simulink subsystem "SimscapePlantModels"  (R2023a)
settings: Solver=VariableStepAuto  StartTime=0.0  StopTime=10.0  RelTol=1e-3
undefined symbols (not defined in the file): AxlFL, AxlFR, AxlRL, AxlRR, EM1, EM2, EM3, EM4, PlntDCDCVoltInit, PlntTrnsfrCaseAxlSpdLock, PlntTrnsfrCaseTrqSplitRatio, ThrmBatt, ThrmBatt1, ThrmBatt2, ThrmBatt3, ThrmBatt4, ThrmEM, ThrmEM1, ThrmEM2, ThrmEM3, ThrmEM4, ThrmPwrE
libraries: fl_lib x30, nesl_utility_internal x13, sdl_lib x3, nesl_utility x2, vehdynlibsens x1
(part 1 of 2)
settings Model: ModifiedByFormat=The MathWorks, Inc.  Creator=The MathWorks, Inc.  LastModifiedBy=The MathWorks, Inc.
settings SolverCC: MaxZcPerStep=1
settings OptimizationCC: ReuseModelBlockBuffer=off
settings DebuggingCC: UnconnectedInputMsg=warning  UnconnectedOutputMsg=warning  UnconnectedLineMsg=warning  SubsystemReferenceDiagnosticForUnitTest=warning
settings ModelReferenceCC: EnableRefExpFcnMdlSchedulingChecks=on
settings RTWCC: DLArmComputeVersion=19.05

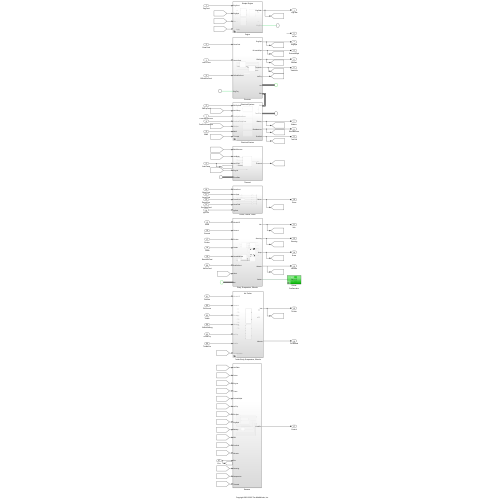
[thumbnail: Simulink's stored preview of the top-level diagram]
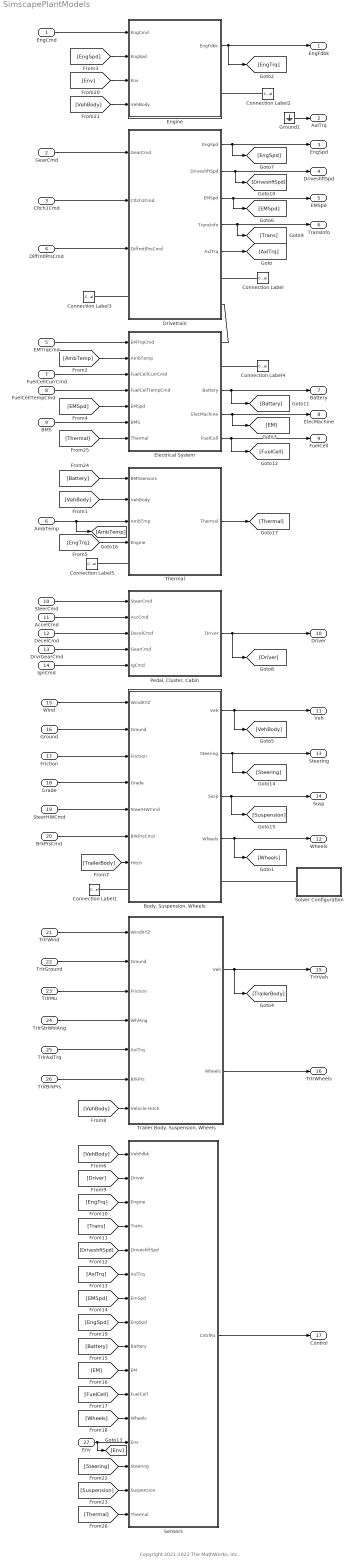
== system SimscapePlantModels ==
  note: Copyright 2021-2022 The MathWorks, Inc.
  EngCmd : Inport
  GearCmd : Inport  Port=2
  Cltch1Cmd : Inport  Port=3
  DiffrntlPrsCmd : Inport  Port=4
  EMTrqCmd : Inport  Port=5
  AmbTemp : Inport  Port=6
  FuelCellCurrCmd : Inport  Port=7
  FuelCellTempCmd : Inport  Port=8
  BMS : Inport  Port=9
  SteerCmd : Inport  Port=10
  AccelCmd : Inport  Port=11
  DecelCmd : Inport  Port=12
  DrvrGearCmd : Inport  Port=13
  IgnCmd : Inport  Port=14
  Wind : Inport  Port=15
  Ground : Inport  Port=16
  Friction : Inport  Port=17
  Grade : Inport  Port=18
  SteerHWCmd : Inport  Port=19
  BrkPrsCmd : Inport  Port=20
  TrlrWind : Inport  Port=21
  TrlrGround : Inport  Port=22
  TrlrMu : Inport  Port=23
  TrlrStrWhlAng : Inport  Port=24
  TrlrAxlTrq : Inport  Port=25
  TrlrBrkPrs : Inport  Port=26
  Env : Inport  Port=27
  "Body, Suspension, Wheels" : Subsystem  VariantControl=Longitudinal Vehicle Dynamics
  Connection Label : ConnectionLabel  Label=Axl
  Connection Label1 : ConnectionLabel  Label=Axl
  Connection Label2 : ConnectionLabel  Label=EngTrq
  Connection Label3 : ConnectionLabel  Label=EngTrq
  Connection Label4 : ConnectionLabel  Label=ThrmElec
  Connection Label5 : ConnectionLabel  Label=ThrmElec
  Drivetrain : Subsystem
  Electrical System : Subsystem  Variant=on  VariantControlMode=label  VariantControl=Choice  LabelModeActiveChoice=Electrical System
      settings: PortSchema="{\"entries\":[{\"content\":{\"sides\":[{\"content\":{\"connectorIds\":[\"In1\",\"In2\",\"In3\",\"In4\",\"In5\",\"In6\",\"In7\"]},\"type\":\"ConnectorPlacement.EquallySpacedRectSide\",\"uuid\":\"168fda7d-02fd-4045-80e4-d70d0b749a9c\"},{\"content\":{\"connectorIds\":[\"RConn1\",\"RConn2\",\"Out1\",\"Out2\",\"Out3\"],\"side\":\"RIGHT\"},\"type\":\"ConnectorPlacement.EquallySpacedRectSide\",\"uuid\":\"a7e9bf4a-b9ce-46d6-8afc-0075c6e03a0c\"},{\"content\":{\"side\":\"TOP\"},\"type\":\"ConnectorPlacement.EquallySpacedRectSide\",\"uuid\":\"81c60468-d7ed-4851-a727-3a9a5b008640\"}]},\"type\":\"ConnectorPlacement.EquallySpacedConnector\",\"uuid\":\"8c7c8f28-264e-479c-b2d0-01b49dca4966\"}],\"packageUris\":[\"http://schema.mathworks.com/mf0/Connector/R2020b\"],\"version\":\"1.0\"}"
  Engine : Subsystem  Variant=on  VariantControlMode=label  LabelModeActiveChoice=Simple Engine
  Ground1 : Ground
  "Pedal, Cluster, Cabin" : Subsystem
  Sensors : Subsystem
  Solver Configuration : Subsystem  Variant=on  VariantControlMode=label  VariantControl=Choice  LabelModeActiveChoice=Solver Configuration
  Thermal : Subsystem
  "Trailer Body, Suspension, Wheels" : Subsystem  Variant=on  VariantControlMode=label  LabelModeActiveChoice=No Trailer
  EngFdbk : Outport
  AxlTrq : Outport  Port=2
  EngSpd : Outport  Port=3
  DriveshftSpd : Outport  Port=4
  EMSpd : Outport  Port=5
  TransInfo : Outport  Port=6
  Battery : Outport  Port=7
  ElecMachine : Outport  Port=8
  FuelCell : Outport  Port=9
  Driver : Outport  Port=10
  Veh : Outport  Port=11
  Wheels : Outport  Port=12
  Steering : Outport  Port=13
  Susp : Outport  Port=14
  TrlrVeh : Outport  Port=15
  TrlrWheels : Outport  Port=16
  Control : Outport  Port=17
  wires:
  Drivetrain/4(TransInfo) -> [Trans], TransInfo/1
  EngCmd/1 -> Engine/1(EngCmd)
  Electrical System/3(FuelCell) -> FuelCell/1, [FuelCell]
  Electrical System/1(Battery) -> Battery/1, [Battery]
  TrlrGround/1 -> "Trailer Body, Suspension, Wheels"/2(Ground)
  Wind/1 -> "Body, Suspension, Wheels"/1(WindXYZ)
  TrlrAxlTrq/1 -> "Trailer Body, Suspension, Wheels"/5(AxlTrq)
  EMTrqCmd/1 -> Electrical System/1(EMTrqCmd)
  DiffrntlPrsCmd/1 -> Drivetrain/3(DiffrntlPrsCmd)
  TrlrMu/1 -> "Trailer Body, Suspension, Wheels"/3(Friction)
  Friction/1 -> "Body, Suspension, Wheels"/3(Friction)
  SteerHWCmd/1 -> "Body, Suspension, Wheels"/5(SteerHWCmd)
  [EMSpd] -> Electrical System/5(EMSpd)
  Ground/1 -> "Body, Suspension, Wheels"/2(Ground)
  SteerCmd/1 -> "Pedal, Cluster, Cabin"/1(SteerCmd)
  TrlrBrkPrs/1 -> "Trailer Body, Suspension, Wheels"/6(BrkPrs)
  Drivetrain/2(DriveshftSpd) -> [DriveshftSpd], DriveshftSpd/1
  "Body, Suspension, Wheels"/1(Veh) -> [VehBody], Veh/1
  Engine/1(EngFdbk) -> [EngTrq], EngFdbk/1
  BrkPrsCmd/1 -> "Body, Suspension, Wheels"/6(BrkPrsCmd)
  Cltch1Cmd/1 -> Drivetrain/2(Cltch1Cmd)
  TrlrWind/1 -> "Trailer Body, Suspension, Wheels"/1(WindXYZ)
  TrlrStrWhlAng/1 -> "Trailer Body, Suspension, Wheels"/4(WhlAng)
  [VehBody] -> "Trailer Body, Suspension, Wheels"/7(Vehicle Hitch)
  "Trailer Body, Suspension, Wheels"/2(Wheels) -> TrlrWheels/1
  Electrical System/2(ElecMachine) -> ElecMachine/1, [EM]
  [TrailerBody] -> "Body, Suspension, Wheels"/7(Hitch)
  DecelCmd/1 -> "Pedal, Cluster, Cabin"/3(DecelCmd)
  DrvrGearCmd/1 -> "Pedal, Cluster, Cabin"/4(GearCmd)
  Drivetrain/3(EMSpd) -> [EMSpd], EMSpd/1
  IgnCmd/1 -> "Pedal, Cluster, Cabin"/5(IgCmd)
  FuelCellTempCmd/1 -> Electrical System/4(FuelCellTempCmd)
  GearCmd/1 -> Drivetrain/1(GearCmd)
  "Body, Suspension, Wheels"/4(Wheels) -> [Wheels], Wheels/1
  "Trailer Body, Suspension, Wheels"/1(Veh) -> TrlrVeh/1, [TrailerBody]
  FuelCellCurrCmd/1 -> Electrical System/3(FuelCellCurrCmd)
  AccelCmd/1 -> "Pedal, Cluster, Cabin"/2(AccCmd)
  Drivetrain/1(EngSpd) -> EngSpd/1, [EngSpd]
  [VehBody] -> Sensors/1(VehFdbk)
  "Pedal, Cluster, Cabin"/1(Driver) -> Driver/1, [Driver]
  [Driver] -> Sensors/2(Driver)
  [EngTrq] -> Sensors/3(Engine)
  [Trans] -> Sensors/4(Trans)
  [DriveshftSpd] -> Sensors/5(DriveshftSpd)
  [AxlTrq] -> Sensors/6(AxlTrq)
  [EMSpd] -> Sensors/7(EmSpd)
  [Battery] -> Sensors/9(Battery)
  [EM] -> Sensors/10(EM)
  [FuelCell] -> Sensors/11(FuelCell)
  [Wheels] -> Sensors/12(Wheels)
  Sensors/1(CntrlRx) -> Control/1
  Env/1 -> [Env], Sensors/13(Env)
  [EngSpd] -> Sensors/8(EngSpd)
  [Env] -> Engine/3(Env)
  [VehBody] -> Engine/4(VehBody)
  [EngSpd] -> Engine/2(EngSpd)
  "Body, Suspension, Wheels"/3(Susp) -> [Suspension], Susp/1
  Grade/1 -> "Body, Suspension, Wheels"/4(Grade)
  Ground1/1 -> AxlTrq/1
  Drivetrain/5(AxlTrq) -> [AxlTrq]
  BMS/1 -> Electrical System/6(BMS)
  [Steering] -> Sensors/14(Steering)
  [Suspension] -> Sensors/15(Suspension)
  "Body, Suspension, Wheels"/2(Steering) -> [Steering], Steering/1
  Thermal/1(Thermal) -> [Thermal]
  [VehBody] -> Thermal/2(VehBody)
  [Battery] -> Thermal/1(BMSSensors)
  [EngTrq] -> Thermal/4(Engine)
  AmbTemp/1 -> [AmbTemp], Thermal/3(AmbTmp)
  [AmbTemp] -> Electrical System/2(AmbTemp)
  [Thermal] -> Electrical System/7(Thermal)
  [Thermal] -> Sensors/16(Thermal)
  connections:
  Connection Label/LConn1 -- Drivetrain/RConn1
  "Body, Suspension, Wheels"/LConn1 -- Connection Label1/LConn1
  Electrical System/RConn1 -- Drivetrain/RConn2
  Drivetrain/LConn1 -- Connection Label3/LConn1
  Connection Label2/LConn1 -- Engine/RConn1
  Solver Configuration/RConn1 -- "Body, Suspension, Wheels"/RConn1
  Thermal/LConn1 -- Connection Label5/LConn1
  Connection Label4/LConn1 -- Electrical System/RConn2

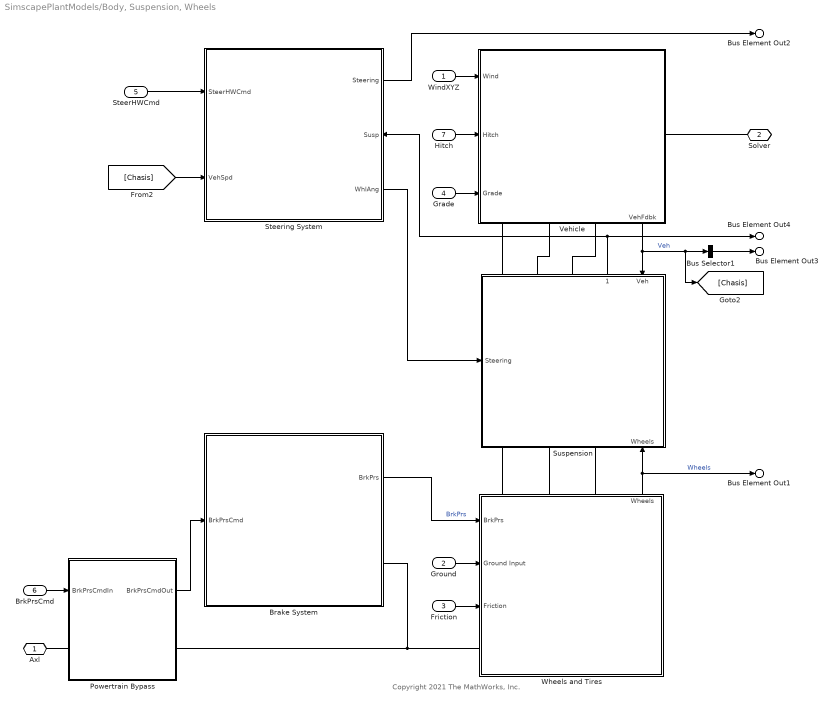
== system SimscapePlantModels/Body, Suspension, Wheels ==
  note: Copyright 2021 The MathWorks, Inc.
  WindXYZ : Inport  Unit=m/s  PortDimensions=3
  Ground : Inport  Port=2  Unit=m  PortDimensions=4
  Friction : Inport  Port=3  Unit=1  PortDimensions=4
  Grade : Inport  Port=4  Unit=deg  PortDimensions=1
  SteerHWCmd : Inport  Port=5  Unit=rad
  BrkPrsCmd : Inport  Port=6  PortDimensions=4
  Hitch : Inport  Port=7
  Brake System : Subsystem  Variant=on  VariantControlMode=label  VariantControl=Choice  LabelModeActiveChoice=Braking Hydraulics and Disc Brakes
      mask Display: image('Caliper.png',[.125,.125,.75,.75])
  Bus Selector1 : BusSelector  OutputSignals=InertFrm,BdyFrm  OutputAsBus=on
  Powertrain Bypass : Subsystem  Variant=on  VariantControlMode=label  VariantControl=Choice  LabelModeActiveChoice=Pass Through
  Steering System : Subsystem  Variant=on  VariantControlMode=label  VariantControl=0  LabelModeActiveChoice=No Steering
      settings: PortSchema="{\"entries\":[{\"content\":{\"sides\":[{\"content\":{\"connectorIds\":[\"In1\",\"In2\"]},\"type\":\"ConnectorPlacement.EquallySpacedRectSide\",\"uuid\":\"f4eae9a1-ee72-4894-9c3f-d81ee40fba89\"},{\"content\":{\"connectorIds\":[\"Out1\",\"In3\",\"Out2\"],\"side\":\"RIGHT\"},\"type\":\"ConnectorPlacement.EquallySpacedRectSide\",\"uuid\":\"c62a78d9-dc5d-4f96-a554-c82d7fa22a9e\"},{\"content\":{\"connectorIds\":[],\"side\":\"TOP\"},\"type\":\"ConnectorPlacement.EquallySpacedRectSide\",\"uuid\":\"38f3851a-1d1e-4a2b-8c09-8e5c8dcc7723\"}]},\"type\":\"ConnectorPlacement.EquallySpacedConnector\",\"uuid\":\"9f269846-92fa-4948-bc2b-71154f41fdde\"}],\"packageUris\":[\"http://schema.mathworks.com/mf0/Connector/R2020b\"],\"version\":\"1.0\"}"
      mask Display:
      | switch get_param(gcb,'ActiveVariant')
      |     case 'Kinematic Steering'
      |         image('KinematicSteering.png');
      |     case 'Mapped Steering'
      |         image('MappedSteering.png');
      |     case 'Dynamic Steering'
      |         image('DynamicSteering.png');
      |     otherwise
      |         image('DynamicSteering.png');
      | end
  Suspension : Subsystem  Variant=on  VariantControlMode=label  VariantControl=Choice  LabelModeActiveChoice=No Suspension
      settings: PortSchema="{\"entries\":[{\"content\":{\"sides\":[{\"content\":{\"connectorIds\":[\"In1\"]},\"type\":\"ConnectorPlacement.EquallySpacedRectSide\",\"uuid\":\"0a9265e3-f55e-4b74-9b74-681dc9522591\"},{\"content\":{\"side\":\"RIGHT\"},\"type\":\"ConnectorPlacement.EquallySpacedRectSide\",\"uuid\":\"92df639a-7bc2-4e90-97ea-0cb216e2f16a\"},{\"content\":{\"connectorIds\":[\"LConn1\",\"LConn2\",\"LConn3\",\"Out1\",\"In2\"],\"side\":\"TOP\"},\"type\":\"ConnectorPlacement.EquallySpacedRectSide\",\"uuid\":\"2064b6cb-c7a8-4cfb-82de-a07750d990cb\"},{\"content\":{\"connectorIds\":[\"RConn1\",\"RConn2\",\"RConn3\",\"In3\"],\"side\":\"BOTTOM\"},\"type\":\"ConnectorPlacement.EquallySpacedRectSide\",\"uuid\":\"169bd4e6-c3fe-4e36-acea-c25875014463\"}]},\"type\":\"ConnectorPlacement.EquallySpacedConnector\",\"uuid\":\"e0b50182-0637-4594-80e7-4ddd0df85797\"}],\"packageUris\":[\"http://schema.mathworks.com/mf0/Connector/R2020b\"],\"version\":\"1.0\"}"
      mask Display:
      | switch get_param(gcb,'ActiveVariant')
      |     case 'Kinematics and Compliance Independent Suspension'
      |         image('KandCSuspension.png');
      |     case 'Kinematics and Compliance Twist Beam Suspension'
      |         image('KandCSuspensionTwistBeam.png');
      |     case 'MacPherson Front Suspension Solid Axle Rear Suspension'
      |         image([imread('suspmacp.png');imread('suspsacoil.png')]);
      |     otherwise
      |         image([imread('suspmacp.png');imread('suspsacoil.png')]);
      | end
  Vehicle : Subsystem  Variant=on  VariantControlMode=label  VariantControl=Choice  LabelModeActiveChoice=Vehicle Body 1DOF Longitudinal
      settings: PortSchema="{\"entries\":[{\"content\":{\"sides\":[{\"content\":{\"connectorIds\":[\"In1\",\"In2\",\"In3\"]},\"type\":\"ConnectorPlacement.EquallySpacedRectSide\",\"uuid\":\"0a9265e3-f55e-4b74-9b74-681dc9522591\"},{\"content\":{\"connectorIds\":[\"RConn1\"],\"side\":\"RIGHT\"},\"type\":\"ConnectorPlacement.EquallySpacedRectSide\",\"uuid\":\"92df639a-7bc2-4e90-97ea-0cb216e2f16a\"},{\"content\":{\"connectorIds\":[],\"side\":\"TOP\"},\"type\":\"ConnectorPlacement.EquallySpacedRectSide\",\"uuid\":\"2064b6cb-c7a8-4cfb-82de-a07750d990cb\"},{\"content\":{\"connectorIds\":[\"RConn2\",\"RConn3\",\"RConn4\",\"Out1\"],\"side\":\"BOTTOM\"},\"type\":\"ConnectorPlacement.EquallySpacedRectSide\",\"uuid\":\"2b34afca-0a88-43db-924f-6476183b84bd\"}]},\"type\":\"ConnectorPlacement.EquallySpacedConnector\",\"uuid\":\"e0b50182-0637-4594-80e7-4ddd0df85797\"}],\"packageUris\":[\"http://schema.mathworks.com/mf0/Connector/R2020b\"],\"version\":\"1.0\"}"
      mask Display: image('6dofcar.png');
  Wheels and Tires : Subsystem  Variant=on  VariantControlMode=label  VariantControl=Choice  LabelModeActiveChoice=MF Tires Longitudinal
      settings: PortSchema="{\"entries\":[{\"content\":{\"sides\":[{\"content\":{\"connectorIds\":[\"In1\",\"In2\",\"In3\",\"LConn1\"]},\"type\":\"ConnectorPlacement.EquallySpacedRectSide\",\"uuid\":\"fdb4d4cd-d0c0-42d9-b073-775af31e96a1\"},{\"content\":{\"connectorIds\":[],\"side\":\"RIGHT\"},\"type\":\"ConnectorPlacement.EquallySpacedRectSide\",\"uuid\":\"04106ddf-9917-4cd4-b177-ae763d642686\"},{\"content\":{\"connectorIds\":[\"LConn2\",\"LConn3\",\"LConn4\",\"Out1\"],\"side\":\"TOP\"},\"type\":\"ConnectorPlacement.EquallySpacedRectSide\",\"uuid\":\"568bf95c-0e25-4c45-a134-c198357b75be\"}]},\"type\":\"ConnectorPlacement.EquallySpacedConnector\",\"uuid\":\"4f44df5e-0d14-43ea-934e-2abe86546e95\"}],\"packageUris\":[\"http://schema.mathworks.com/mf0/Connector/R2020b\"],\"version\":\"1.0\"}"
      mask Display: image('wheel3dof.png')
  Axl : PMIOPort  Side=Left
  Solver : PMIOPort  Port=2  Side=Right
  Bus Element Out3 : Outport  PortName=Veh
  Bus Element Out2 : Outport  Port=2  PortName=Steering
  Bus Element Out4 : Outport  Port=3  PortName=Susp
  Bus Element Out1 : Outport  Port=4  PortName=Wheels
  wires:
  SteerHWCmd/1 -> Steering System/1(SteerHWCmd)
  Bus Selector1/1 -> Bus Element Out3/1
  WindXYZ/1 -> Vehicle/1(Wind)
  Brake System/1(BrkPrs) -> Wheels and Tires/1(BrkPrs)  "BrkPrs"
  Steering System/2(WhlAng) -> Suspension/1(Steering)
  Suspension/1(SuspChassis) -> Bus Element Out4/1, Steering System/3(Susp)
  Powertrain Bypass/1(BrkPrsCmdOut) -> Brake System/1(BrkPrsCmd)
  Wheels and Tires/1(Wheels) -> Bus Element Out1/1, Suspension/3(Wheels)  "Wheels"
  Grade/1 -> Vehicle/3(Grade)
  Hitch/1 -> Vehicle/2(Hitch)
  Friction/1 -> Wheels and Tires/3(Friction)
  Steering System/1(Steering) -> Bus Element Out2/1
  [Chasis] -> Steering System/2(VehSpd)
  Ground/1 -> Wheels and Tires/2(Ground Input)
  Vehicle/1(VehFdbk) -> [Chasis], Bus Selector1/1, Suspension/2(Veh)  "Veh"
  BrkPrsCmd/1 -> Powertrain Bypass/1(BrkPrsCmdIn)
  connections:
  Brake System/RConn1 -- Powertrain Bypass/RConn1 -- Wheels and Tires/LConn1
  Vehicle/RConn2 -- Suspension/LConn1
  Vehicle/RConn3 -- Suspension/LConn2
  Vehicle/RConn4 -- Suspension/LConn3
  Wheels and Tires/LConn2 -- Suspension/RConn1
  Wheels and Tires/LConn3 -- Suspension/RConn2
  Wheels and Tires/LConn4 -- Suspension/RConn3
  Vehicle/RConn1 -- Solver/RConn1
  Axl/RConn1 -- Powertrain Bypass/LConn1

== system SimscapePlantModels/Drivetrain ==
  note: Copyright 2018-2021 The MathWorks, Inc.
  GearCmd : Inport
  Cltch1Cmd : Inport  Port=2
  DiffrntlPrsCmd : Inport  Port=3
  Drivetrain Layout : Subsystem  VariantControl=New
      settings: PortSchema="{\"entries\":[{\"content\":{\"sides\":[{\"content\":{\"connectorIds\":[\"LConn1\",\"In1\"]},\"type\":\"ConnectorPlacement.EquallySpacedRectSide\",\"uuid\":\"aca18566-8f68-4dbe-a1ea-7891e9b0f8a0\"},{\"content\":{\"connectorIds\":[\"Out1\",\"Out2\",\"RConn1\"],\"side\":\"RIGHT\"},\"type\":\"ConnectorPlacement.EquallySpacedRectSide\",\"uuid\":\"80817b32-8ae2-43ef-bc82-fae1c7a772cb\"},{\"content\":{\"connectorIds\":[],\"side\":\"TOP\"},\"type\":\"ConnectorPlacement.EquallySpacedRectSide\",\"uuid\":\"fadb27fa-7a73-4d3f-b69d-888e371ed2d5\"}]},\"type\":\"ConnectorPlacement.EquallySpacedConnector\",\"uuid\":\"7287b0c1-67df-44d5-bf90-b5b5a04fa161\"}],\"packageUris\":[\"http://schema.mathworks.com/mf0/Connector/R2020b\"],\"version\":\"1.0\"}"
  Transmission and Actuators : Subsystem  Variant=on  VariantControlMode=label  LabelModeActiveChoice=Conventional Vehicle
  EngTrq : PMIOPort  Side=Left
  Axl : PMIOPort  Port=2  Side=Right
  EM : PMIOPort  Port=3  Side=Right
  EngSpd : Outport  Unit=rad/s  VectorParamsAs1DForOutWhenUnconnected=off
  DriveshftSpd : Outport  Port=2  VectorParamsAs1DForOutWhenUnconnected=off
  EMSpd : Outport  Port=3  Unit=rad/s  VectorParamsAs1DForOutWhenUnconnected=off
  TransInfo : Outport  Port=4  VectorParamsAs1DForOutWhenUnconnected=off
  AxlTrq : Outport  Port=5  VectorParamsAs1DForOutWhenUnconnected=off
  wires:
  Transmission and Actuators/1(Info) -> TransInfo/1  "TransInfo"
  DiffrntlPrsCmd/1 -> Drivetrain Layout/1(DiffrntlPrsCmd)
  Cltch1Cmd/1 -> Transmission and Actuators/2(Cltch1Cmd)
  Drivetrain Layout/1(DriveshftSpd) -> DriveshftSpd/1
  GearCmd/1 -> Transmission and Actuators/1(GearCmd)
  Transmission and Actuators/2(EngSpd) -> EngSpd/1
  Transmission and Actuators/3(EMSpd) -> EMSpd/1
  Drivetrain Layout/2(AxlTrq) -> AxlTrq/1
  connections:
  Transmission and Actuators/LConn2 -- EM/RConn1
  Drivetrain Layout/RConn1 -- Axl/RConn1
  Drivetrain Layout/LConn1 -- Transmission and Actuators/RConn1
  Transmission and Actuators/LConn1 -- EngTrq/RConn1

== system SimscapePlantModels/Electrical System ==
  EMTrqCmd : Inport
  AmbTemp : Inport  Port=2
  FuelCellCurrCmd : Inport  Port=3
  FuelCellTempCmd : Inport  Port=4
  EMSpd : Inport  Port=5
  BMS : Inport  Port=6
  Thermal : Inport  Port=7
  Electrical System : Subsystem  VariantControl=Electrical System
  Electrical System 1EM : Subsystem  VariantControl=Electrical System 1EM
  Electrical System 2EM : Subsystem  VariantControl=Electrical System 2EM
  Fuel Cell Electrical System : Subsystem  VariantControl=Fuel Cell Electrical System  ReferencedSubsystem=FuelCellElectricSystem
  No Electrification : Subsystem  VariantControl=No Electrification  ReferencedSubsystem=NoElectrical
  EM : PMIOPort  Side=Right
  ThrmElec : PMIOPort  Port=2  Side=Right
  Battery : Outport
  ElecMachine : Outport  Port=2
  FuelCell : Outport  Port=3

== system SimscapePlantModels/Engine ==
  EngCmd : Inport
  EngSpd : Inport  Port=2
  Env : Inport  Port=3
  VehBody : Inport  Port=4
  FMU Engine : Subsystem  VariantControl=FMU Engine  ReferencedSubsystem=FMUEngineSSC
  No Engine : Subsystem  VariantControl=No Engine  ReferencedSubsystem=NoEngine
  Simple Engine : Subsystem  VariantControl=Simple Engine  ReferencedSubsystem=SimpleEngineSSC
  EngTrq : PMIOPort  Side=Right
  EngFdbk : Outport  VectorParamsAs1DForOutWhenUnconnected=off

== system SimscapePlantModels/Pedal, Cluster, Cabin ==
  SteerCmd : Inport
  AccCmd : Inport  Port=2
  DecelCmd : Inport  Port=3
  GearCmd : Inport  Port=4
  IgCmd : Inport  Port=5
  Brake Pedal : Subsystem
  Bus Creator1 : BusCreator  Inputs=5
  Dead Zone2 : DeadZone  LowerValue=0  UpperValue=.01  ZeroCross=off
  Dead Zone3 : DeadZone  LowerValue=-.01  UpperValue=.01  ZeroCross=off
  Signal Specification : SignalSpecification  Unit=rad
  Signal Specification{1..4} (4 alike) : SignalSpecification  Unit=1
  Driver : Outport
  wires:
  Dead Zone3/1 -> Signal Specification/1
  Signal Specification1/1 -> Bus Creator1/2  "AccelFdbk"
  Signal Specification4/1 -> Bus Creator1/5  "IgnFdbk"
  Brake Pedal/1(DecelFdbk) -> Signal Specification2/1
  Signal Specification/1 -> Bus Creator1/1  "SteerFdbk"
  Signal Specification2/1 -> Bus Creator1/3  "DecelFdbk"
  GearCmd/1 -> Signal Specification3/1
  Bus Creator1/1 -> Driver/1
  IgCmd/1 -> Signal Specification4/1
  Signal Specification3/1 -> Bus Creator1/4  "GearFdbk"
  Dead Zone2/1 -> Signal Specification1/1
  SteerCmd/1 -> Dead Zone3/1
  AccCmd/1 -> Dead Zone2/1
  DecelCmd/1 -> Brake Pedal/1(DecelCmd)

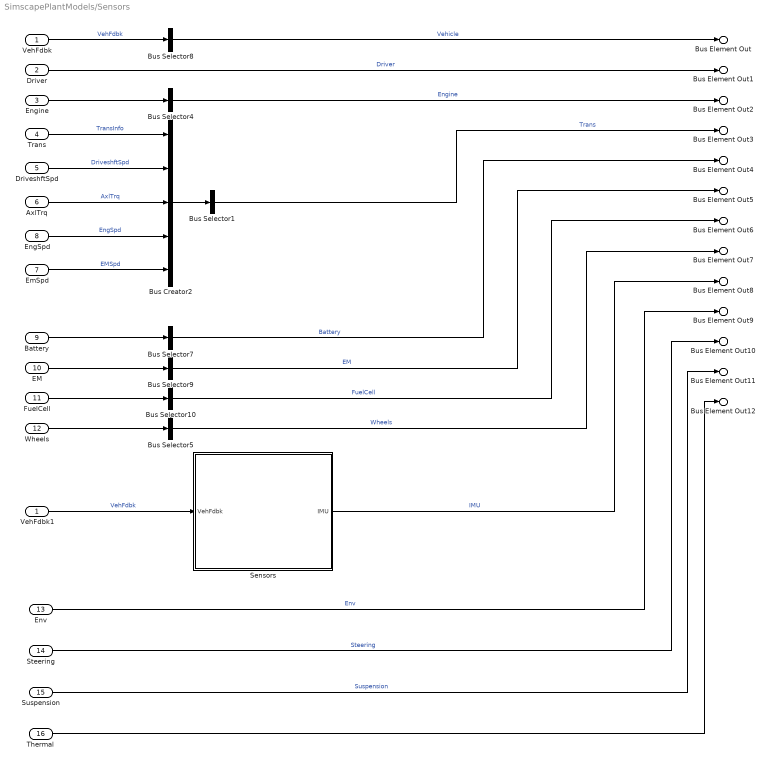
== system SimscapePlantModels/Sensors ==
  VehFdbk : Inport
  Driver : Inport  Port=2
  Engine : Inport  Port=3
  Trans : Inport  Port=4
  DriveshftSpd : Inport  Port=5
  AxlTrq : Inport  Port=6
  EmSpd : Inport  Port=7
  EngSpd : Inport  Port=8
  Battery : Inport  Port=9
  EM : Inport  Port=10
  FuelCell : Inport  Port=11
  Wheels : Inport  Port=12
  Env : Inport  Port=13
  Steering : Inport  Port=14
  Suspension : Inport  Port=15
  Thermal : Inport  Port=16
  Bus Creator2 : BusCreator  Inputs=5
  Bus Selector1 : BusSelector  OutputSignals=TransInfo.Cltch1State,TransInfo.Cltch2State,DriveshftSpd,AxlTrq,EngSpd,EMSpd,TransInfo.TransInfo.Trans.TransGear  OutputAsBus=on
  Bus Selector10 : BusSelector  OutputSignals=FuelCellVolt,FuelCellCurr,H2Flw  OutputAsBus=on
  Bus Selector4 : BusSelector  OutputSignals=EngTrq,Map,Mat,ThrPosPct,WgAreaPct,IntkCamPhase,ExhCamPhase,TurboRackPos,EgrVlvAreaPct,VarCompRatioPos,IntkVlvLift,VarIntkRunLen,Afr,IntkSwirlVlvPos,TurboSpd,Iat,Ect,EgrVlvDeltaPrs,EgrVlvInTemp  OutputAsBus=on
  Bus Selector5 : BusSelector  OutputSignals=Wheels.BrkPrs,Wheels.Kappa,Wheels.Alpha,Wheels.Omega  OutputAsBus=on
  Bus Selector7 : BusSelector  OutputSignals=BattSoc,BattVolt,BattCurr,BattPwr,BMSSensors  OutputAsBus=on
  Bus Selector8 : BusSelector  OutputSignals=BdyFrm.Cg.Vel.xdot,BdyFrm.Cg.Acc.xddot  OutputAsBus=on
  Bus Selector9 : BusSelector  OutputSignals=EMTrq,EMPwrElec  OutputAsBus=on
  Sensors : Subsystem  Variant=on  VariantControlMode=label  VariantControl=Choice  LabelModeActiveChoice=No IMU Sensor
  VehFdbk1 : InportShadow
  Bus Element Out : Outport  PortName=CntrlRx  Element=Vehicle
  Bus Element Out1 : Outport  PortName=CntrlRx  Element=Driver
  Bus Element Out2 : Outport  PortName=CntrlRx  Element=Engine
  Bus Element Out3 : Outport  PortName=CntrlRx  Element=Trans
  Bus Element Out4 : Outport  PortName=CntrlRx  Element=Battery
  Bus Element Out5 : Outport  PortName=CntrlRx  Element=EM
  Bus Element Out6 : Outport  PortName=CntrlRx  Element=FuelCell
  Bus Element Out7 : Outport  PortName=CntrlRx  Element=Wheels
  Bus Element Out8 : Outport  PortName=CntrlRx  Element=IMU
  Bus Element Out9 : Outport  PortName=CntrlRx  Element=Env
  Bus Element Out10 : Outport  PortName=CntrlRx  Element=Steering
  Bus Element Out11 : Outport  PortName=CntrlRx  Element=Suspension
  Bus Element Out12 : Outport  PortName=CntrlRx  Element=Thermal
  wires:
  Bus Selector1/1 -> Bus Element Out3/1  "Trans"
  Bus Creator2/1 -> Bus Selector1/1
  Trans/1 -> Bus Creator2/1  "TransInfo"
  EngSpd/1 -> Bus Creator2/4  "EngSpd"
  Env/1 -> Bus Element Out9/1  "Env"
  Driver/1 -> Bus Element Out1/1  "Driver"
  Sensors/1(IMU) -> Bus Element Out8/1  "IMU"
  VehFdbk1/1 -> Sensors/1(VehFdbk)  "VehFdbk"
  Wheels/1 -> Bus Selector5/1
  FuelCell/1 -> Bus Selector10/1
  EM/1 -> Bus Selector9/1
  Battery/1 -> Bus Selector7/1
  EmSpd/1 -> Bus Creator2/5  "EMSpd"
  AxlTrq/1 -> Bus Creator2/3  "AxlTrq"
  DriveshftSpd/1 -> Bus Creator2/2  "DriveshftSpd"
  Engine/1 -> Bus Selector4/1
  VehFdbk/1 -> Bus Selector8/1  "VehFdbk"
  Bus Selector4/1 -> Bus Element Out2/1  "Engine"
  Bus Selector10/1 -> Bus Element Out6/1  "FuelCell"
  Bus Selector9/1 -> Bus Element Out5/1  "EM"
  Bus Selector8/1 -> Bus Element Out/1  "Vehicle"
  Bus Selector7/1 -> Bus Element Out4/1  "Battery"
  Bus Selector5/1 -> Bus Element Out7/1  "Wheels"
  Steering/1 -> Bus Element Out10/1  "Steering"
  Suspension/1 -> Bus Element Out11/1  "Suspension"
  Thermal/1 -> Bus Element Out12/1

== system SimscapePlantModels/Solver Configuration ==
  Local Solver : nesl_utility/Solver Configuration  VariantControl=Local Solver  PhysicalDomain=network_engine_domain  SubClassName=solver  LeftPortType=input  RightPortType=generic  Tones=[]  Harmonics=[]  SimulateNoise=off  Profile=off  UseLocalSampling=off  EnableSwitchedLinearOptims=on  FrequencyDomain=off  UseCCode=off  RelTol=0.001  AbsTol=0.001  MinStep=1e-09  ToWorkspace=off  RevertToSquareIcSolve=off  NumHomotopyIterations=100  PhasorMode=off  PhasorModeNumHarmonics=1  ConsistencySolver=NEWTON_XTOL_AFTER_FTOL  IndexReductionMethod=DerivativeReplacement  DoDC=off  ResidualTolerance=1e-09  ConsistencyTolSource=LOCAL  ConsistencyAbsTol=0.001  ConsistencyRelTol=0.001  ConsistencyTolFactor=0.001  UseLocalSolver=on  LocalSolverChoice=NE_BACKWARD_EULER_ADVANCER  ResolveIndetEquations=on  FunctionEvalNumThread=1  LocalSolverSampleTime=0.1  DoFixedCost=on  MaxNonlinIter=3  MaxModeIter=2  ComputeImpulses=off  ImpulseIterations=2  LinearAlgebra=auto  LinearAlgebraNumThread=0  EquationFormulation=NE_TIME_EF  DelaysMemoryBudget=1024  AutomaticFiltering=on  FilteringTimeConstant=0.001  PartitionStorageMethod=AS_NEEDED  PartitionMemoryBudget=1024  PartitionMethod=ROBUST
  Solver Configuration : nesl_utility/Solver Configuration  VariantControl=Solver Configuration  PhysicalDomain=network_engine_domain  SubClassName=solver  LeftPortType=input  RightPortType=generic  Tones=[]  Harmonics=[]  SimulateNoise=off  Profile=off  UseLocalSampling=off  EnableSwitchedLinearOptims=on  FrequencyDomain=off  UseCCode=off  RelTol=0.001  AbsTol=0.001  MinStep=1e-09  ToWorkspace=off  RevertToSquareIcSolve=off  NumHomotopyIterations=100  PhasorMode=off  PhasorModeNumHarmonics=1  ConsistencySolver=NEWTON_XTOL_AFTER_FTOL  IndexReductionMethod=DerivativeReplacement  DoDC=off  ResidualTolerance=1e-09  ConsistencyTolSource=LOCAL  ConsistencyAbsTol=0.001  ConsistencyRelTol=0.001  ConsistencyTolFactor=0.001  UseLocalSolver=off  LocalSolverChoice=NE_BACKWARD_EULER_ADVANCER  ResolveIndetEquations=on  FunctionEvalNumThread=1  LocalSolverSampleTime=0.001  DoFixedCost=off  MaxNonlinIter=3  MaxModeIter=2  ComputeImpulses=off  ImpulseIterations=2  LinearAlgebra=auto  LinearAlgebraNumThread=0  EquationFormulation=NE_TIME_EF  DelaysMemoryBudget=1024  AutomaticFiltering=on  FilteringTimeConstant=0.001  PartitionStorageMethod=AS_NEEDED  PartitionMemoryBudget=1024  PartitionMethod=ROBUST
  a : PMIOPort  Side=Right

== system SimscapePlantModels/Thermal ==
  BMSSensors : Inport
  VehBody : Inport  Port=2
  AmbTmp : Inport  Port=3
  Engine : Inport  Port=4
  Electrical Cooling : Subsystem  Variant=on  VariantControlMode=label  LabelModeActiveChoice=No Thermal Effect
  Terminator : Terminator
  ThrmElec : PMIOPort  Side=Left
  Thermal : Outport
  wires:
  AmbTmp/1 -> Electrical Cooling/3(AmbTmp)
  VehBody/1 -> Electrical Cooling/2(VehBody)
  BMSSensors/1 -> Electrical Cooling/1(BMSSensors)
  Electrical Cooling/1(Thermal) -> Thermal/1
  Engine/1 -> Terminator/1
  connections:
  ThrmElec/RConn1 -- Electrical Cooling/LConn1

== system SimscapePlantModels/Trailer Body, Suspension, Wheels ==
  WindXYZ : Inport
  Ground : Inport  Port=2
  Friction : Inport  Port=3
  WhlAng : Inport  Port=4
  AxlTrq : Inport  Port=5
  BrkPrs : Inport  Port=6
  Vehicle Hitch : Inport  Port=7
  No Trailer : Subsystem  VariantControl=No Trailer
  One-Axle Trailer : Subsystem  VariantControl=One-Axle Trailer  ReferencedSubsystem=OneAxleTrailer
  Veh : Outport  VectorParamsAs1DForOutWhenUnconnected=off
  Wheels : Outport  Port=2  VectorParamsAs1DForOutWhenUnconnected=off

== system SimscapePlantModels/Body, Suspension, Wheels/Brake System ==
  BrkPrsCmd : Inport
  Braking Hydraulics and Disc Brakes : Subsystem  VariantControl=Braking Hydraulics and Disc Brakes  ReferencedSubsystem=BrakingHydraulicsDiscBrakesSSC
  Axl : PMIOPort  Side=Right
  BrkPrs : Outport

== system SimscapePlantModels/Body, Suspension, Wheels/Powertrain Bypass ==
  BrkPrsCmdIn : Inport
  External Signal Source : Subsystem  VariantControl=External Signal Source
  Pass Through : Subsystem  VariantControl=Pass Through
  AxlTrqIn : PMIOPort  Side=Left
  AxlTrqOut : PMIOPort  Port=2  Side=Right
  BrkPrsCmdOut : Outport

== system SimscapePlantModels/Body, Suspension, Wheels/Steering System ==
  SteerHWCmd : Inport
  VehSpd : Inport  Port=2
  Susp : Inport  Port=3
  No Steering : Subsystem  VariantControl=No Steering  ReferencedSubsystem=NoSteering
  Steering : Outport
  WhlAng : Outport  Port=2  VectorParamsAs1DForOutWhenUnconnected=off

== system SimscapePlantModels/Body, Suspension, Wheels/Suspension ==
  Steering : Inport
  Veh : Inport  Port=2
  Wheels : Inport  Port=3
  No Suspension : Subsystem  VariantControl=No Suspension  ReferencedSubsystem=NoSuspensionSSC
  SuspVeh : PMIOPort  Side=Left
  FrntAxlVeh : PMIOPort  Port=2  Side=Left
  RearAxlVeh : PMIOPort  Port=3  Side=Left
  SuspWhl : PMIOPort  Port=4  Side=Right
  FrntAxlWhl : PMIOPort  Port=5  Side=Right
  RearAxlWhl : PMIOPort  Port=6  Side=Right
  SuspChassis : Outport

== system SimscapePlantModels/Body, Suspension, Wheels/Vehicle ==
  Wind : Inport
  Hitch : Inport  Port=2
  Grade : Inport  Port=3
  Vehicle Body 1DOF Longitudinal : Subsystem  VariantControl=Vehicle Body 1DOF Longitudinal  ReferencedSubsystem=VehicleBody1DOFLongitudinalSSC
  Vehicle Body 3DOF Longitudinal : Subsystem  VariantControl=Vehicle Body 3DOF Longitudinal  ReferencedSubsystem=VehicleBody3DOFLongitudinalSSC
  Solver : PMIOPort  Side=Right
  SuspVeh : PMIOPort  Port=2  Side=Right
  FrntAxlVeh : PMIOPort  Port=3  Side=Right
  RearAxlVeh : PMIOPort  Port=4  Side=Right
  VehFdbk : Outport

== system SimscapePlantModels/Body, Suspension, Wheels/Wheels and Tires ==
  BrkPrs : Inport
  Ground Input : Inport  Port=2
  Friction : Inport  Port=3
  MF Tires Longitudinal : Subsystem  VariantControl=MF Tires Longitudinal  ReferencedSubsystem=MFTiresLongitudinalSSC
  Axl : PMIOPort  Side=Left
  SuspWhl : PMIOPort  Port=2  Side=Left
  FrntAxlWhl : PMIOPort  Port=3  Side=Left
  RearAxlWhl : PMIOPort  Port=4  Side=Left
  Wheels : Outport

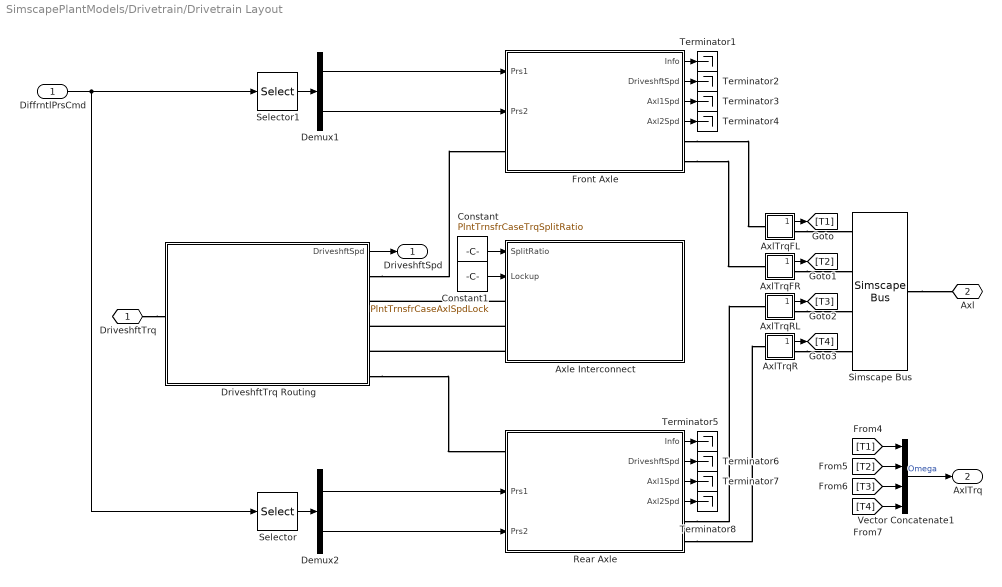
== system SimscapePlantModels/Drivetrain/Drivetrain Layout ==
  DiffrntlPrsCmd : Inport
  AxlTrqFL : Subsystem
  AxlTrqFR : Subsystem
  AxlTrqR : Subsystem
  AxlTrqRL : Subsystem
  Axle Interconnect : Subsystem  Variant=on  VariantControlMode=label  VariantControl=Choice  LabelModeActiveChoice=No Interconnect
  Constant : Constant  Value=PlntTrnsfrCaseTrqSplitRatio  SampleTime=-1
  Constant1 : Constant  Value=PlntTrnsfrCaseAxlSpdLock  SampleTime=-1
  Demux1 : Demux  Outputs=2
  Demux2 : Demux  Outputs=2
  DriveshftTrq Routing : Subsystem  Variant=on  VariantControlMode=label  VariantControl=Choice  LabelModeActiveChoice=One Actuator FWD
  Front Axle : Subsystem  Variant=on  VariantControlMode=label  VariantControl=Choice  LabelModeActiveChoice=Open Differential
  Rear Axle : Subsystem  Variant=on  VariantControlMode=label  VariantControl=Choice  LabelModeActiveChoice=No Differential
      settings: PortSchema="{\"entries\":[{\"content\":{\"sides\":[{\"content\":{\"connectorIds\":[\"LConn1\",\"In1\",\"In2\"]},\"type\":\"ConnectorPlacement.EquallySpacedRectSide\",\"uuid\":\"74f8b1d8-6b3a-4eeb-b984-715de40eb708\"},{\"content\":{\"connectorIds\":[\"Out1\",\"Out2\",\"Out3\",\"Out4\",\"RConn1\",\"RConn2\"],\"side\":\"RIGHT\"},\"type\":\"ConnectorPlacement.EquallySpacedRectSide\",\"uuid\":\"c00021b1-b8b4-4ff3-9b35-429da9caaad3\"},{\"content\":{\"connectorIds\":[],\"side\":\"TOP\"},\"type\":\"ConnectorPlacement.EquallySpacedRectSide\",\"uuid\":\"0bf4e327-a693-4202-b285-43d08d42df4d\"}]},\"type\":\"ConnectorPlacement.EquallySpacedConnector\",\"uuid\":\"b41f4b2c-0e15-48ba-ac2c-145a8c4b8844\"}],\"packageUris\":[\"http://schema.mathworks.com/mf0/Connector/R2020b\"],\"version\":\"1.0\"}"
  Selector : Selector  InputPortWidth=4  IndexOptions=Index vector (dialog)  Indices=[3 4]  OutputSizes=1
  Selector1 : Selector  InputPortWidth=4  IndexOptions=Index vector (dialog)  Indices=[1 2]  OutputSizes=1
  Simscape Bus : SimscapeBus  HierarchyStrings=AxlFL;AxlFR;AxlRL;AxlRR
  Terminator{1..8} (8 alike) : Terminator
  Vector Concatenate1 : Concatenate  NumInputs=4
  DriveshftTrq : PMIOPort  Side=Left
  Axl : PMIOPort  Port=2  Side=Right
  DriveshftSpd : Outport  VectorParamsAs1DForOutWhenUnconnected=off
  AxlTrq : Outport  Port=2  VectorParamsAs1DForOutWhenUnconnected=off
  wires:
  Selector/1 -> Demux2/1
  Demux1/2 -> Front Axle/2(Prs2)
  Demux1/1 -> Front Axle/1(Prs1)
  Selector1/1 -> Demux1/1
  DiffrntlPrsCmd/1 -> Selector1/1, Selector/1
  Rear Axle/1(Info) -> Terminator5/1
  Front Axle/1(Info) -> Terminator1/1
  Demux2/1 -> Rear Axle/1(Prs1)
  Demux2/2 -> Rear Axle/2(Prs2)
  Front Axle/2(DriveshftSpd) -> Terminator2/1
  Front Axle/3(Axl1Spd) -> Terminator3/1
  Front Axle/4(Axl2Spd) -> Terminator4/1
  Rear Axle/2(DriveshftSpd) -> Terminator6/1
  Rear Axle/3(Axl1Spd) -> Terminator7/1
  Rear Axle/4(Axl2Spd) -> Terminator8/1
  Constant/1 -> Axle Interconnect/1(SplitRatio)
  Constant1/1 -> Axle Interconnect/2(Lockup)
  [T4] -> Vector Concatenate1/4
  [T3] -> Vector Concatenate1/3
  [T2] -> Vector Concatenate1/2
  Vector Concatenate1/1 -> AxlTrq/1  "Omega"
  [T1] -> Vector Concatenate1/1
  AxlTrqFL/1(Trq) -> [T1]
  AxlTrqFR/1(Trq) -> [T2]
  AxlTrqRL/1(Trq) -> [T3]
  AxlTrqR/1(Trq) -> [T4]
  DriveshftTrq Routing/1(DriveshftSpd) -> DriveshftSpd/1
  connections:
  Simscape Bus/RConn1 -- Axl/RConn1
  Front Axle/RConn1 -- AxlTrqFL/LConn1
  Front Axle/RConn2 -- AxlTrqFR/LConn1
  Rear Axle/RConn2 -- AxlTrqR/LConn1
  Rear Axle/RConn1 -- AxlTrqRL/LConn1
  DriveshftTrq Routing/RConn1 -- Front Axle/LConn1
  DriveshftTrq Routing/RConn5 -- Rear Axle/LConn1
  Axle Interconnect/LConn1 -- DriveshftTrq Routing/RConn2
  Axle Interconnect/LConn2 -- DriveshftTrq Routing/RConn3
  Axle Interconnect/LConn3 -- DriveshftTrq Routing/RConn4
  AxlTrqFL/RConn1 -- Simscape Bus/LConn1
  AxlTrqFR/RConn1 -- Simscape Bus/LConn2
  AxlTrqRL/RConn1 -- Simscape Bus/LConn3
  AxlTrqR/RConn1 -- Simscape Bus/LConn4
  DriveshftTrq/RConn1 -- DriveshftTrq Routing/LConn1

== system SimscapePlantModels/Drivetrain/Transmission and Actuators ==
  GearCmd : Inport
  Cltch1Cmd : Inport  Port=2
  Conventional Vehicle : Subsystem  VariantControl=Conventional Vehicle
  Electric Vehicle 1EM : Subsystem  VariantControl=Electric Vehicle 1EM  ReferencedSubsystem=BEV1EMSSC
  Electric Vehicle 2EM : Subsystem  VariantControl=Electric Vehicle 2EM  ReferencedSubsystem=BEV2EMSSC
  Electric Vehicle 3EM : Subsystem  VariantControl=Electric Vehicle 3EM  ReferencedSubsystem=BEV3EMSSC
  Electric Vehicle 4EM : Subsystem  VariantControl=Electric Vehicle 4EM  ReferencedSubsystem=BEV4EMSSC
  Hybrid Electric Vehicle IPS : Subsystem  VariantControl=Hybrid Electric Vehicle IPS  ReferencedSubsystem=HEVIPSSSC
  Hybrid Electric Vehicle MM : Subsystem  VariantControl=Hybrid Electric Vehicle MM  ReferencedSubsystem=HEVMMSSC
  Hybrid Electric Vehicle P0 : Subsystem  VariantControl=Hybrid Electric Vehicle P0  ReferencedSubsystem=HEVP0SSC
  Hybrid Electric Vehicle P1 : Subsystem  VariantControl=Hybrid Electric Vehicle P1  ReferencedSubsystem=HEVP1SSC
  Hybrid Electric Vehicle P2 : Subsystem  VariantControl=Hybrid Electric Vehicle P2  ReferencedSubsystem=HEVP2SSC
  Hybrid Electric Vehicle P3 : Subsystem  VariantControl=Hybrid Electric Vehicle P3  ReferencedSubsystem=HEVP3SSC
  Hybrid Electric Vehicle P4 : Subsystem  VariantControl=Hybrid Electric Vehicle P4  ReferencedSubsystem=HEVP4SSC
  EngTrq : PMIOPort  Side=Left
  EM : PMIOPort  Port=2  Side=Left
  DriveshftTrq : PMIOPort  Port=3  Side=Right
  Info : Outport  VectorParamsAs1DForOutWhenUnconnected=off
  EngSpd : Outport  Port=2  VectorParamsAs1DForOutWhenUnconnected=off
  EMSpd : Outport  Port=3  VectorParamsAs1DForOutWhenUnconnected=off  BusOutputAsStruct=on

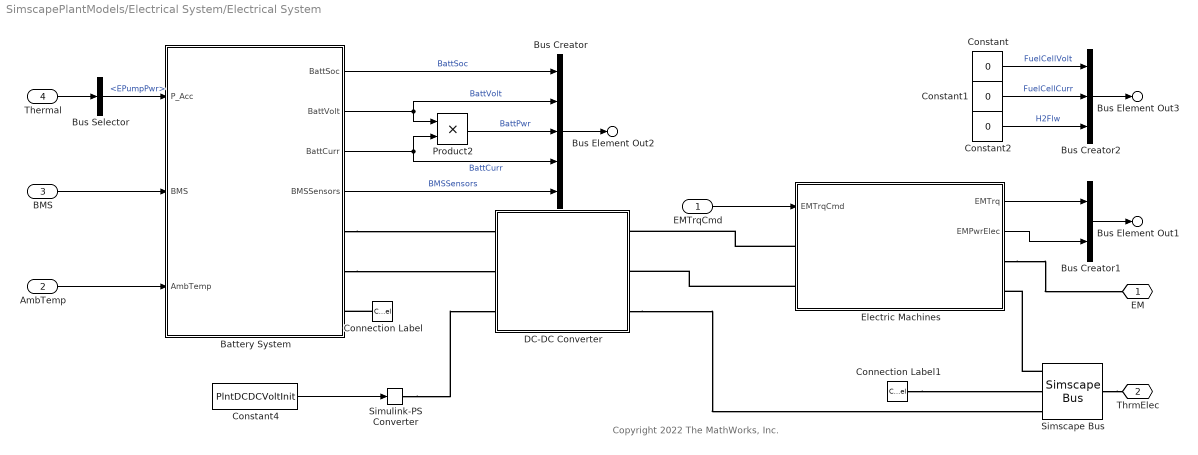
== system SimscapePlantModels/Electrical System/Electrical System ==
  note: Copyright 2022 The MathWorks, Inc.
  EMTrqCmd : Inport
  AmbTemp : Inport  Port=2
  BMS : Inport  Port=3
  Thermal : Inport  Port=4
  Battery System : Subsystem  Variant=on  VariantControlMode=label  LabelModeActiveChoice=Mapped Battery
  Bus Creator : BusCreator  Inputs=5
  Bus Creator1 : BusCreator  Inputs=2
  Bus Creator2 : BusCreator  Inputs=3
  Bus Selector : BusSelector  OutputSignals=EPumpPwr
  Connection Label : ConnectionLabel  Label=ThrmBatt
  Connection Label1 : ConnectionLabel  Label=ThrmBatt
  Constant : Constant  Value=0  SampleTime=-1
  Constant1 : Constant  Value=0  SampleTime=-1
  Constant2 : Constant  Value=0  SampleTime=-1
  Constant4 : Constant  Value=PlntDCDCVoltInit  SampleTime=-1
  DC-DC Converter : Subsystem  Variant=on  VariantControlMode=label  VariantControl=Choice  LabelModeActiveChoice=DC-DC Converter
  Electric Machines : Subsystem  Variant=on  VariantControlMode=label  VariantControl=Choice  LabelModeActiveChoice=1EM
  Product2 : Product
  Simscape Bus : SimscapeBus  HierarchyStrings=ThrmEM;ThrmBatt;ThrmPwrE
  Simulink-PS Converter : nesl_utility_internal/Simulink-PS Converter  PhysicalDomain=network_engine_domain  SubClassName=ps_input  LeftPortType=input  RightPortType=output  PseudoPeriodic=off  Frequencies=[]  NoiseDistribution=none  NoiseParameters=[]  Unit=1  AffineConversion=off  FilteringAndDerivatives=provide  SimscapeFilterOrder=1  InputFilterTimeConstant=0.001  UdotUserProvided=0
  EM : PMIOPort  Side=Right
  ThrmElec : PMIOPort  Port=2  Side=Right
  Bus Element Out2 : Outport  PortName=Battery
  Bus Element Out1 : Outport  Port=2  PortName=ElecMachine
  Bus Element Out3 : Outport  Port=3  PortName=FuelCell
  wires:
  Electric Machines/2(EMPwrElec) -> Bus Creator1/2
  Electric Machines/1(EMTrq) -> Bus Creator1/1
  EMTrqCmd/1 -> Electric Machines/1(EMTrqCmd)
  Battery System/4(BMSSensors) -> Bus Creator/5  "BMSSensors"
  AmbTemp/1 -> Battery System/3(AmbTemp)
  BMS/1 -> Battery System/2(BMS)
  Constant4/1 -> Simulink-PS Converter/1
  Product2/1 -> Bus Creator/3  "BattPwr"
  Battery System/1(BattSoc) -> Bus Creator/1  "BattSoc"
  Battery System/3(BattCurr) -> Product2/2, Bus Creator/4  "BattCurr"
  Battery System/2(BattVolt) -> Bus Creator/2, Product2/1  "BattVolt"
  Bus Creator/1 -> Bus Element Out2/1
  Constant1/1 -> Bus Creator2/2  "FuelCellCurr"
  Constant2/1 -> Bus Creator2/3  "H2Flw"
  Bus Creator1/1 -> Bus Element Out1/1
  Bus Creator2/1 -> Bus Element Out3/1
  Constant/1 -> Bus Creator2/1  "FuelCellVolt"
  Bus Selector/1 -> Battery System/1(P_Acc)  "<EPumpPwr>"
  Thermal/1 -> Bus Selector/1
  connections:
  Electric Machines/RConn1 -- EM/RConn1
  Electric Machines/LConn2 -- DC-DC Converter/RConn2
  Electric Machines/LConn1 -- DC-DC Converter/RConn1
  Battery System/RConn2 -- DC-DC Converter/LConn2
  Battery System/RConn1 -- DC-DC Converter/LConn1
  Simulink-PS Converter/RConn1 -- DC-DC Converter/LConn3
  DC-DC Converter/RConn3 -- Simscape Bus/LConn3
  Simscape Bus/RConn1 -- ThrmElec/RConn1
  Connection Label/LConn1 -- Battery System/RConn3
  Connection Label1/LConn1 -- Simscape Bus/LConn2
  Simscape Bus/LConn1 -- Electric Machines/RConn2

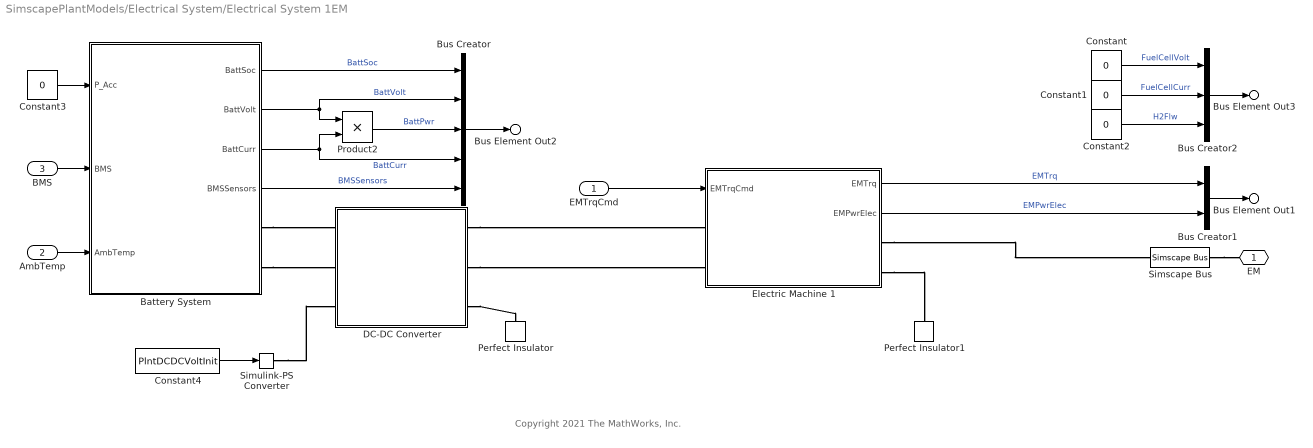
== system SimscapePlantModels/Electrical System/Electrical System 1EM ==
  note: Copyright 2021 The MathWorks, Inc.
  EMTrqCmd : Inport
  AmbTemp : Inport  Port=2
  BMS : Inport  Port=3
  Battery System : Subsystem  Variant=on  VariantControlMode=label  LabelModeActiveChoice=Mapped Battery
  Bus Creator : BusCreator  Inputs=5
  Bus Creator1 : BusCreator  Inputs=2
  Bus Creator2 : BusCreator  Inputs=3
  Constant{,1..3} (4 alike) : Constant  Value=0  SampleTime=-1
  Constant4 : Constant  Value=PlntDCDCVoltInit  SampleTime=-1
  DC-DC Converter : Subsystem  Variant=on  VariantControlMode=label  VariantControl=Choice  LabelModeActiveChoice=DC-DC Converter
  Electric Machine 1 : Subsystem  Variant=on  VariantControlMode=label  LabelModeActiveChoice=Mapped EM
  Perfect Insulator : fl_lib/Thermal/Thermal Elements/Perfect Insulator  T_specify=off  T_priority=None  T=293.15 K  T_nominal_specify=off  T_nominal_unit=K  T_nominal_value=1
  Perfect Insulator1 : fl_lib/Thermal/Thermal Elements/Perfect Insulator  T_specify=off  T_priority=None  T=293.15 K  T_nominal_specify=off  T_nominal_unit=K  T_nominal_value=1
  Product2 : Product
  Simscape Bus : SimscapeBus  HierarchyStrings=EM1
  Simulink-PS Converter : nesl_utility_internal/Simulink-PS Converter  PhysicalDomain=network_engine_domain  SubClassName=ps_input  LeftPortType=input  RightPortType=output  PseudoPeriodic=off  Frequencies=[]  NoiseDistribution=none  NoiseParameters=[]  Unit=1  AffineConversion=off  FilteringAndDerivatives=provide  SimscapeFilterOrder=1  InputFilterTimeConstant=0.001  UdotUserProvided=0
  EM : PMIOPort  Side=Right
  Bus Element Out2 : Outport  PortName=Battery
  Bus Element Out1 : Outport  Port=2  PortName=ElecMachine
  Bus Element Out3 : Outport  Port=3  PortName=FuelCell
  wires:
  Constant3/1 -> Battery System/1(P_Acc)
  Constant/1 -> Bus Creator2/1  "FuelCellVolt"
  Bus Creator2/1 -> Bus Element Out3/1
  Bus Creator1/1 -> Bus Element Out1/1
  Constant2/1 -> Bus Creator2/3  "H2Flw"
  Constant1/1 -> Bus Creator2/2  "FuelCellCurr"
  Bus Creator/1 -> Bus Element Out2/1
  Battery System/2(BattVolt) -> Bus Creator/2, Product2/1  "BattVolt"
  Battery System/3(BattCurr) -> Bus Creator/4, Product2/2  "BattCurr"
  Battery System/1(BattSoc) -> Bus Creator/1  "BattSoc"
  Product2/1 -> Bus Creator/3  "BattPwr"
  EMTrqCmd/1 -> Electric Machine 1/1(EMTrqCmd)
  Electric Machine 1/1(EMTrq) -> Bus Creator1/1  "EMTrq"
  Electric Machine 1/2(EMPwrElec) -> Bus Creator1/2  "EMPwrElec"
  Constant4/1 -> Simulink-PS Converter/1
  BMS/1 -> Battery System/2(BMS)
  AmbTemp/1 -> Battery System/3(AmbTemp)
  Battery System/4(BMSSensors) -> Bus Creator/5  "BMSSensors"
  connections:
  Electric Machine 1/RConn1 -- Simscape Bus/LConn1
  Electric Machine 1/RConn2 -- Perfect Insulator1/LConn1
  DC-DC Converter/RConn3 -- Perfect Insulator/LConn1
  DC-DC Converter/RConn2 -- Electric Machine 1/LConn2
  DC-DC Converter/RConn1 -- Electric Machine 1/LConn1
  Simscape Bus/RConn1 -- EM/RConn1
  Simulink-PS Converter/RConn1 -- DC-DC Converter/LConn3
  Battery System/RConn1 -- DC-DC Converter/LConn1
  Battery System/RConn2 -- DC-DC Converter/LConn2

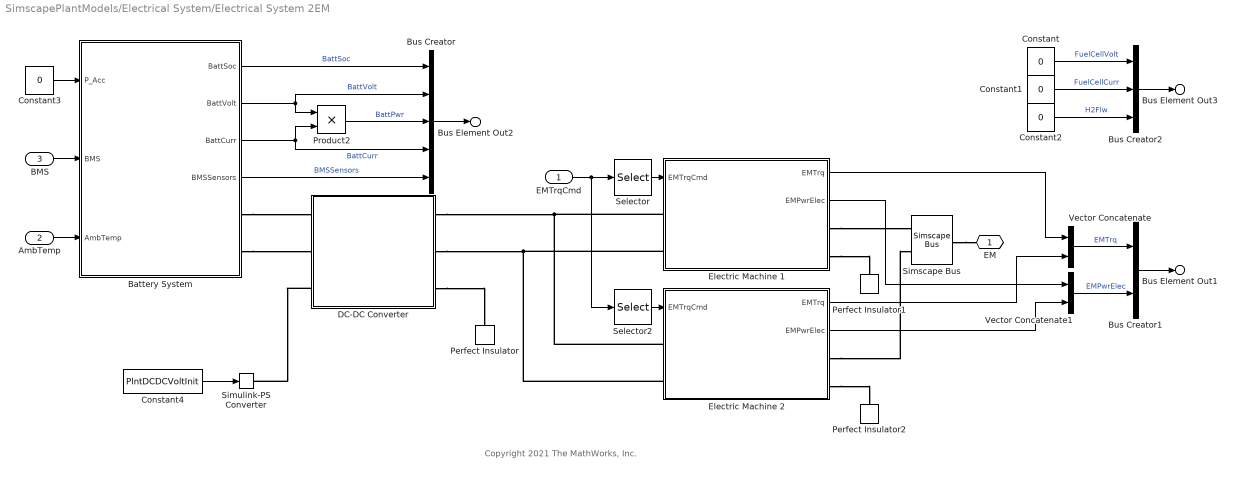
== system SimscapePlantModels/Electrical System/Electrical System 2EM ==
  note: Copyright 2021 The MathWorks, Inc.
  EMTrqCmd : Inport
  AmbTemp : Inport  Port=2
  BMS : Inport  Port=3
  Battery System : Subsystem  Variant=on  VariantControlMode=label  LabelModeActiveChoice=Mapped Battery
  Bus Creator : BusCreator  Inputs=5
  Bus Creator1 : BusCreator  Inputs=2
  Bus Creator2 : BusCreator  Inputs=3
  Constant{,1..3} (4 alike) : Constant  Value=0  SampleTime=-1
  Constant4 : Constant  Value=PlntDCDCVoltInit  SampleTime=-1
  DC-DC Converter : Subsystem  Variant=on  VariantControlMode=label  VariantControl=Choice  LabelModeActiveChoice=DC-DC Converter
  Electric Machine 1 : Subsystem  Variant=on  VariantControlMode=label  LabelModeActiveChoice=Mapped EM
  Electric Machine 2 : Subsystem  Variant=on  VariantControlMode=label  LabelModeActiveChoice=Mapped EM
  Perfect Insulator : fl_lib/Thermal/Thermal Elements/Perfect Insulator  T_specify=off  T_priority=None  T=293.15 K  T_nominal_specify=off  T_nominal_unit=K  T_nominal_value=1
  Perfect Insulator1 : fl_lib/Thermal/Thermal Elements/Perfect Insulator  T_specify=off  T_priority=None  T=293.15 K  T_nominal_specify=off  T_nominal_unit=K  T_nominal_value=1
  Perfect Insulator2 : fl_lib/Thermal/Thermal Elements/Perfect Insulator  T_specify=off  T_priority=None  T=293.15 K  T_nominal_specify=off  T_nominal_unit=K  T_nominal_value=1
  Product2 : Product
  Selector : Selector  InputPortWidth=2  IndexOptions=Index vector (dialog)  Indices=[1]  OutputSizes=1
  Selector2 : Selector  InputPortWidth=2  IndexOptions=Index vector (dialog)  Indices=[2]  OutputSizes=1
  Simscape Bus : SimscapeBus  HierarchyStrings=EM1;EM2
  Simulink-PS Converter : nesl_utility_internal/Simulink-PS Converter  PhysicalDomain=network_engine_domain  SubClassName=ps_input  LeftPortType=input  RightPortType=output  PseudoPeriodic=off  Frequencies=[]  NoiseDistribution=none  NoiseParameters=[]  Unit=1  AffineConversion=off  FilteringAndDerivatives=provide  SimscapeFilterOrder=1  InputFilterTimeConstant=0.001  UdotUserProvided=0
  Vector Concatenate : Concatenate
  Vector Concatenate1 : Concatenate
  EM : PMIOPort  Side=Right
  Bus Element Out2 : Outport  PortName=Battery
  Bus Element Out1 : Outport  Port=2  PortName=ElecMachine
  Bus Element Out3 : Outport  Port=3  PortName=FuelCell
  wires:
  Electric Machine 1/2(EMPwrElec) -> Vector Concatenate1/1
  Constant/1 -> Bus Creator2/1  "FuelCellVolt"
  Bus Creator2/1 -> Bus Element Out3/1
  Bus Creator1/1 -> Bus Element Out1/1
  Constant2/1 -> Bus Creator2/3  "H2Flw"
  Constant1/1 -> Bus Creator2/2  "FuelCellCurr"
  Electric Machine 1/1(EMTrq) -> Vector Concatenate/1
  Electric Machine 2/2(EMPwrElec) -> Vector Concatenate1/2
  Electric Machine 2/1(EMTrq) -> Vector Concatenate/2
  Selector/1 -> Electric Machine 1/1(EMTrqCmd)
  Selector2/1 -> Electric Machine 2/1(EMTrqCmd)
  EMTrqCmd/1 -> Selector2/1, Selector/1
  Vector Concatenate/1 -> Bus Creator1/1  "EMTrq"
  Vector Concatenate1/1 -> Bus Creator1/2  "EMPwrElec"
  Constant4/1 -> Simulink-PS Converter/1
  Constant3/1 -> Battery System/1(P_Acc)
  AmbTemp/1 -> Battery System/3(AmbTemp)
  BMS/1 -> Battery System/2(BMS)
  Battery System/4(BMSSensors) -> Bus Creator/5  "BMSSensors"
  Battery System/2(BattVolt) -> Bus Creator/2, Product2/1  "BattVolt"
  Product2/1 -> Bus Creator/3  "BattPwr"
  Battery System/1(BattSoc) -> Bus Creator/1  "BattSoc"
  Bus Creator/1 -> Bus Element Out2/1
  Battery System/3(BattCurr) -> Bus Creator/4, Product2/2  "BattCurr"
  connections:
  Electric Machine 1/RConn1 -- Simscape Bus/LConn1
  Electric Machine 1/RConn2 -- Perfect Insulator1/LConn1
  DC-DC Converter/RConn3 -- Perfect Insulator/LConn1
  Electric Machine 1/LConn2 -- Electric Machine 2/LConn2 -- DC-DC Converter/RConn2
  Electric Machine 1/LConn1 -- Electric Machine 2/LConn1 -- DC-DC Converter/RConn1
  Electric Machine 2/RConn1 -- Simscape Bus/LConn2
  Simscape Bus/RConn1 -- EM/RConn1
  Electric Machine 2/RConn2 -- Perfect Insulator2/LConn1
  DC-DC Converter/LConn3 -- Simulink-PS Converter/RConn1
  Battery System/RConn1 -- DC-DC Converter/LConn1
  Battery System/RConn2 -- DC-DC Converter/LConn2

== system SimscapePlantModels/Pedal, Cluster, Cabin/Brake Pedal ==
  DecelCmd : Inport
  Dead Zone1 : DeadZone  Commented=through  LowerValue=0  UpperValue=.01  ZeroCross=off
  DecelFdbk : Outport
  wires:
  Dead Zone1/1 -> DecelFdbk/1
  DecelCmd/1 -> Dead Zone1/1

== system SimscapePlantModels/Sensors/Sensors ==
  VehFdbk : Inport
  IMU Sensor : Subsystem  VariantControl=IMU Sensor
  No IMU Sensor : Subsystem  VariantControl=No IMU Sensor
  IMU : Outport

== system SimscapePlantModels/Thermal/Electrical Cooling ==
  BMSSensors : Inport
  VehBody : Inport  Port=2
  AmbTmp : Inport  Port=3
  Electrical Cooling System : Subsystem  VariantControl=Electrical Cooling System  ReferencedSubsystem=ElectricalCoolingSystemSSC
  No Thermal Effect : Subsystem  VariantControl=No Thermal Effect
  ThrmElec : PMIOPort  Side=Left
  Thermal : Outport

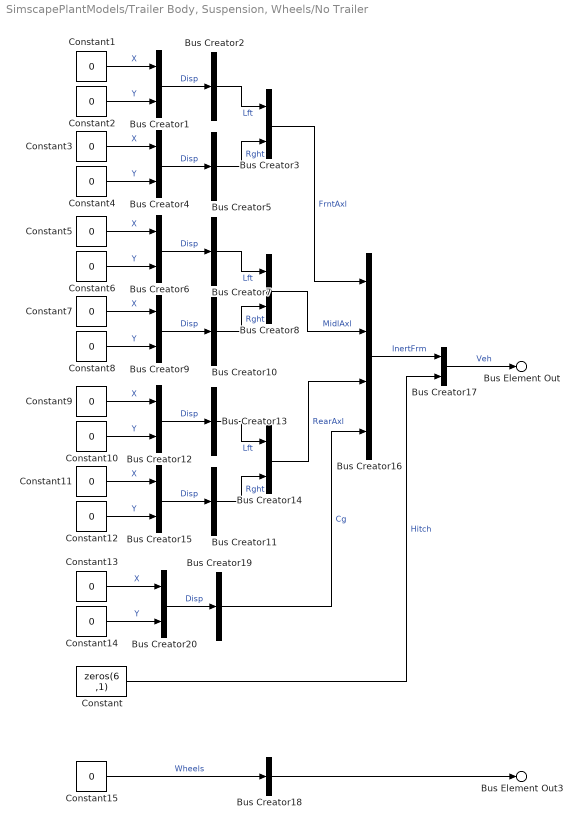
== system SimscapePlantModels/Trailer Body, Suspension, Wheels/No Trailer ==
  Bus Creator{1,3..4,6,8..9,12,14..15,17,20} (11 alike) : BusCreator  Inputs=2
  Bus Creator{2,5,7,10..11,13,18..19} (8 alike) : BusCreator  Inputs=1
  Bus Creator16 : BusCreator  Inputs=4
  Constant : Constant  Value=zeros(6 ,1)  SampleTime=-1
  Constant{1..15} (15 alike) : Constant  Value=0  SampleTime=-1
  Bus Element Out3 : Outport  PortName=Wheels
  Bus Element Out : Outport  Port=2  PortName=Veh
  wires:
  Constant1/1 -> Bus Creator1/1  "X"
  Bus Creator18/1 -> Bus Element Out3/1
  Constant2/1 -> Bus Creator1/2  "Y"
  Bus Creator1/1 -> Bus Creator2/1  "Disp"
  Bus Creator4/1 -> Bus Creator5/1  "Disp"
  Constant4/1 -> Bus Creator4/2  "Y"
  Constant3/1 -> Bus Creator4/1  "X"
  Bus Creator5/1 -> Bus Creator3/2  "Rght"
  Bus Creator2/1 -> Bus Creator3/1  "Lft"
  Bus Creator7/1 -> Bus Creator8/1  "Lft"
  Bus Creator10/1 -> Bus Creator8/2  "Rght"
  Constant7/1 -> Bus Creator9/1  "X"
  Constant8/1 -> Bus Creator9/2  "Y"
  Bus Creator9/1 -> Bus Creator10/1  "Disp"
  Bus Creator6/1 -> Bus Creator7/1  "Disp"
  Constant6/1 -> Bus Creator6/2  "Y"
  Constant5/1 -> Bus Creator6/1  "X"
  Constant9/1 -> Bus Creator12/1  "X"
  Constant10/1 -> Bus Creator12/2  "Y"
  Bus Creator12/1 -> Bus Creator13/1  "Disp"
  Bus Creator15/1 -> Bus Creator11/1  "Disp"
  Constant12/1 -> Bus Creator15/2  "Y"
  Constant11/1 -> Bus Creator15/1  "X"
  Bus Creator11/1 -> Bus Creator14/2  "Rght"
  Bus Creator13/1 -> Bus Creator14/1  "Lft"
  Bus Creator8/1 -> Bus Creator16/2  "MidlAxl"
  Bus Creator14/1 -> Bus Creator16/3  "RearAxl"
  Bus Creator3/1 -> Bus Creator16/1  "FrntAxl"
  Bus Creator16/1 -> Bus Creator17/1  "InertFrm"
  Bus Creator17/1 -> Bus Element Out/1  "Veh"
  Constant15/1 -> Bus Creator18/1  "Wheels"
  Bus Creator19/1 -> Bus Creator16/4  "Cg"
  Constant13/1 -> Bus Creator20/1  "X"
  Constant14/1 -> Bus Creator20/2  "Y"
  Bus Creator20/1 -> Bus Creator19/1  "Disp"
  Constant/1 -> Bus Creator17/2  "Hitch"
